simulink model "operate_flexible_link"  (R2023a)
settings: Solver=ode1  StartTime=0.0  StopTime=100  FixedStep=1/30  RelTol=1e-3  EnableMultiTasking=on
undefined symbols (not defined in the file or in its folder): HIL
libraries: quarc_library x5
settings Model: SimulationMode=external  TunableVars=pos  TunableVarsStorageClass=Auto  Creator=kentaroohki  LastModifiedBy=Flexible4
settings SolverCC: AlgebraicLoopSolver=TrustRegion  PositivePriorityOrder=on
settings DataIOCC: SaveOperatingPoint=on  SaveFormat=Structure  SaveOutput=off  SignalLogging=off  DSMLogging=off  InspectSignalLogs=on  SaveTime=off  ReturnWorkspaceOutputs=off
settings OptimizationCC: OptimizeBlockIOStorage=off  InitFltsAndDblsToZero=on  EfficientMapNaN2IntZero=off  BufferReusableBoundary=off
settings DebuggingCC: UnconnectedInputMsg=warning  UnconnectedOutputMsg=warning  UnconnectedLineMsg=warning  ArithmeticOperatorsInVariantConditions=warning
settings ModelReferenceCC: EnableRefExpFcnMdlSchedulingChecks=on
settings SFSimCC: SimUseLocalCustomCode=off  CustomCodeUndefinedFunction=UseInterfaceOnly
settings RTWCC: Description=QUARC Win64 Target Using Toolchain  SystemTargetFile=quarc_win64.tlc  TemplateMakefile=quarc_default_tmf  RTWUseLocalCustomCode=off  Toolchain=QUARC win64 | nmake (64-bit Windows)  BuildConfiguration=Debug
settings STFCustomTargetCC: SystemTargetFile=quarc_win64.tlc
settings GRTTargetCC: ParMdlRefBuildCompliant=off  CompOptLevelCompliant=off  CombineOutputUpdateFcns=off  MatFileLogging=off  CPPClassGenCompliant=off  GRTInterface=on  ExtMode=on  ExtModeMexFile=quarc_comm

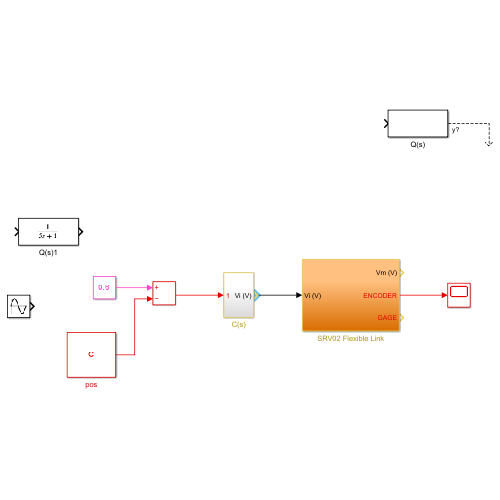
[thumbnail: Simulink's stored preview of the top-level diagram]
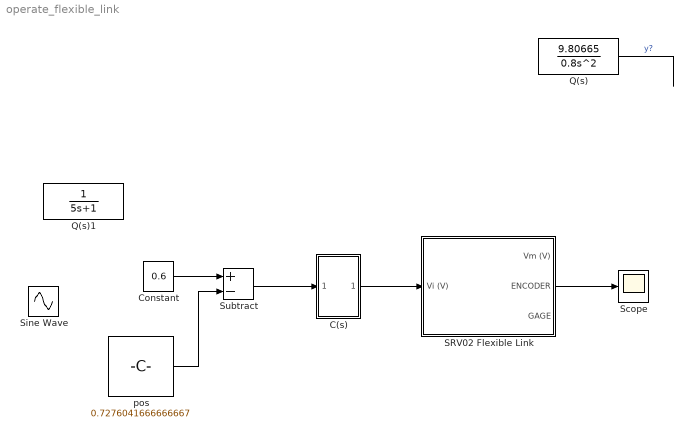
== system operate_flexible_link ==
  C(s) : Subsystem
  Constant : Constant  Value=0.6  OutDataTypeStr=double
  Q(s) : TransferFcn  Numerator=[9.80665]  Denominator=[0.8 0 0]
  Q(s)1 : TransferFcn  Denominator=[5 1]
  SRV02 Flexible Link : Subsystem
  Scope : Scope
  Sine Wave : Sin  SampleTime=0
  Subtract : Sum  Inputs=+-  AccumDataTypeStr=double
  pos : Constant  Value=0.7276041666666667  OutDataTypeStr=double  SampleTime=1/30
  wires:
  Q(s)/1 -> ?  "y?"
  SRV02 Flexible Link/2(ENCODER) -> Scope/1
  Subtract/1 -> C(s)/1(In1)
  C(s)/1(Vi (V)) -> SRV02 Flexible Link/1(Vi (V))
  pos/1 -> Subtract/2
  Constant/1 -> Subtract/1

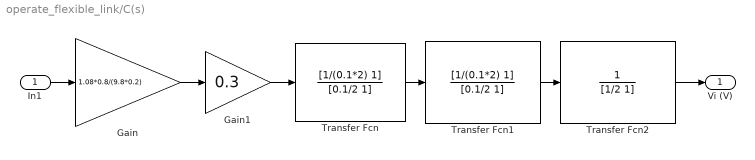
== system operate_flexible_link/C(s) ==
  In1 : Inport
  Gain : Gain  Gain=1.08*0.8/(9.8*0.2)
  Gain1 : Gain  Gain=0.3
  Transfer Fcn : TransferFcn  Numerator=[1/(0.1*2) 1]  Denominator=[0.1/2 1]
  Transfer Fcn1 : TransferFcn  Numerator=[1/(0.1*2) 1]  Denominator=[0.1/2 1]
  Transfer Fcn2 : TransferFcn  Denominator=[1/2 1]
  Vi (V) : Outport
  wires:
  Transfer Fcn/1 -> Transfer Fcn1/1
  Gain/1 -> Gain1/1
  In1/1 -> Gain/1
  Gain1/1 -> Transfer Fcn/1
  Transfer Fcn1/1 -> Transfer Fcn2/1
  Transfer Fcn2/1 -> Vi (V)/1

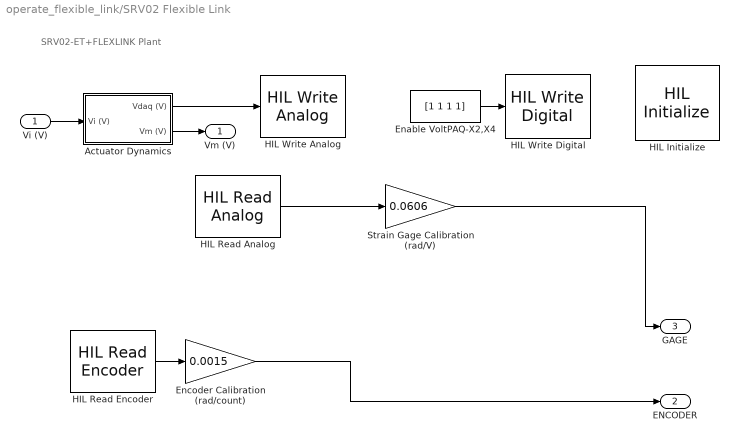
== system operate_flexible_link/SRV02 Flexible Link ==
  note: SRV02-ET+FLEXLINK Plant
  Vi (V) : Inport
  Actuator Dynamics : Subsystem
  Enable VoltPAQ-X2,X4 : Constant  Value=[1 1 1 1]
  Encoder Calibration (rad/count) : Gain  Gain=0.0015  SaturateOnIntegerOverflow=on  OutDataTypeStr=Inherit: Same as input  ParamDataTypeStr=Inherit: Same as input
  HIL Initialize : quarc_library/Data Acquisition/Generic/Configuration/HIL Initialize  object_name=HIL-1  board_type=q2_usb  board_number=0  board_options=d0=digital;d1=digital;led=auto;update_rate=normal  exclusive=off  active=off  hardware_clocks=[0:2]  clock_modes=[]  initial_clock_frequencies=[]  set_clock_params_at_start=off  set_clock_params_at_switch_in=off  set_clock_frequencies_at_start=off  set_clock_frequencies_at_switch_in=off  analog_input_channels=[0:1]  analog_input_configurations=[]  analog_input_maximums=10  analog_input_minimums=-10  set_analog_input_params_at_start=on  set_analog_input_params_at_switch_in=off  analog_output_channels=[0:1]  analog_output_maximums=10  analog_output_minimums=-10  initial_analog_outputs=[0]  final_analog_outputs=[0]  watchdog_analog_outputs=0  set_analog_output_params_at_start=on  set_analog_output_params_at_switch_in=off  set_analog_outputs_at_start=on  set_analog_outputs_at_switch_in=off  set_analog_outputs_at_terminate=on  set_analog_outputs_at_switch_out=off  set_analog_outputs_on_watchdog=off  digital_input_channels=[]  digital_output_channels=[0:7]  digital_output_configuration=[]  initial_digital_outputs=[0]  final_digital_outputs=[0]  watchdog_digital_outputs=[0]  set_digital_output_params_at_start=off  set_digital_output_params_at_switch_in=off  set_digital_outputs_at_start=on  set_digital_outputs_at_switch_in=off  set_digital_outputs_at_terminate=on  set_digital_outputs_at_switch_out=off  set_digital_outputs_on_watchdog=off  encoder_channels=[0:1]  quadrature=[4]  encoder_filter_frequency=[]  initial_encoder_counts=[0]  set_encoder_params_at_start=on  set_encoder_params_at_switch_in=off  set_encoder_counts_at_start=on  set_encoder_counts_at_switch_in=off  pwm_channels=[]  pwm_modes=[0]  pwm_frequency=1/0.020  pwm_configuration=[]  pwm_alignment=[]  pwm_polarity=[]  pwm_leading_deadband=[]  pwm_trailing_deadband=[]  initial_pwm_outputs=[0]  final_pwm_outputs=[0]  watchdog_pwm_outputs=[0]  set_pwm_params_at_start=on  set_pwm_params_at_switch_in=off  set_pwm_outputs_at_start=on  set_pwm_outputs_at_switch_in=off  set_pwm_outputs_at_terminate=on  set_pwm_outputs_at_switch_out=off  set_pwm_outputs_on_watchdog=off  other_output_channels=[]  initial_other_outputs=[]  final_other_outputs=[]  watchdog_other_outputs=[]  set_other_outputs_at_start=off  set_other_outputs_at_switch_in=off  set_other_outputs_at_terminate=off  set_other_outputs_at_switch_out=off  set_other_outputs_on_watchdog=off
  HIL Read Analog : quarc_library/Data Acquisition/Generic/Immediate I//O/HIL Read Analog  object_name=HIL-1  channels=0  sample_time=qc_get_step_size  active=on  vector_output=off
  HIL Read Encoder : quarc_library/Data Acquisition/Generic/Immediate I//O/HIL Read Encoder  object_name=HIL-1  channels=0  sample_time=qc_get_step_size  active=on  vector_output=off  data_type_mode=Inherit via back propagation  data_type=double
  HIL Write Analog : quarc_library/Data Acquisition/Generic/Immediate I//O/HIL Write Analog  object_name=HIL-1  channels=0  sample_time=-1  active=off  vector_input=off
  HIL Write Digital : quarc_library/Data Acquisition/Generic/Immediate I//O/HIL Write Digital  object_name=HIL-1  channels=[0:3]  sample_time=-1  active=off  vector_input=on
      settings: SourceProductName=QUARC Targets
  Strain Gage Calibration (rad/V) : Gain  Gain=0.0606  SaturateOnIntegerOverflow=on  OutDataTypeStr=Inherit: Same as input  ParamDataTypeStr=Inherit: Same as input
  Vm (V) : Outport  InitialOutput=0  VectorParamsAs1DForOutWhenUnconnected=off
  ENCODER : Outport  Port=2  InitialOutput=0  VectorParamsAs1DForOutWhenUnconnected=off
  GAGE : Outport  Port=3  InitialOutput=0  VectorParamsAs1DForOutWhenUnconnected=off
  wires:
  Encoder Calibration (rad/count)/1 -> ENCODER/1
  Actuator Dynamics/2(Vm (V)) -> Vm (V)/1
  Actuator Dynamics/1(Vdaq (V)) -> HIL Write Analog/1
  Vi (V)/1 -> Actuator Dynamics/1(Vi (V))
  Enable VoltPAQ-X2,X4/1 -> HIL Write Digital/1
  HIL Read Analog/1 -> Strain Gage Calibration (rad/V)/1
  Strain Gage Calibration (rad/V)/1 -> GAGE/1
  HIL Read Encoder/1 -> Encoder Calibration (rad/count)/1

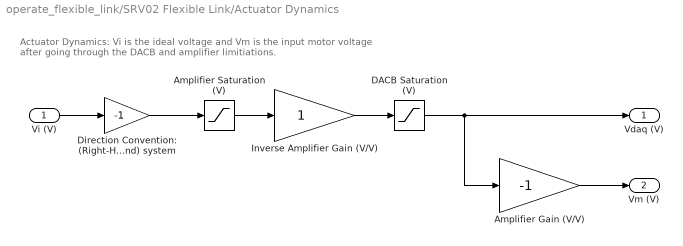
== system operate_flexible_link/SRV02 Flexible Link/Actuator Dynamics ==
  note: Actuator Dynamics: Vi is the ideal voltage and Vm is the
      | input motor voltage after going through the DACB and amplifier limitiations.
  Vi (V) : Inport
  Amplifier Saturation (V) : Saturate  UpperLimit=24  LowerLimit=-24
  Amplifier Gain (V/V) : Gain  Gain=-1
  DACB Saturation (V) : Saturate  UpperLimit=10  LowerLimit=-10
  Direction Convention: (Right-Hand) system : Gain  Gain=-1  SaturateOnIntegerOverflow=on  OutDataTypeStr=Inherit: Same as input  ParamDataTypeStr=Inherit: Same as input
  Inverse Amplifier Gain (V/V) : Gain
  Vdaq (V) : Outport  VectorParamsAs1DForOutWhenUnconnected=off
  Vm (V) : Outport  Port=2  VectorParamsAs1DForOutWhenUnconnected=off
  wires:
  Direction Convention: (Right-Hand) system/1 -> Amplifier Saturation (V)/1
  Amplifier Gain (V/V)/1 -> Vm (V)/1
  DACB Saturation (V)/1 -> Vdaq (V)/1, Amplifier Gain (V/V)/1
  Inverse Amplifier Gain (V/V)/1 -> DACB Saturation (V)/1
  Amplifier Saturation (V)/1 -> Inverse Amplifier Gain (V/V)/1
  Vi (V)/1 -> Direction Convention: (Right-Hand) system/1
